simulink model "RWCday13experimentsPWM"  (R2023a)
settings: Solver=ode45  StartTime=0.0  StopTime=100  MaxStep=0.01  RelTol=1e-3
model workspace (MAT data in the model file):
  J = Simulink.Parameter
  J.Value = [0.0067  0  0; 0  0.033  0; 0  0  0.033]
  J.DataType = 'auto'
  J.Complexity = 'real'
  J.Dimensions = [3 3]
  Jscinv = Simulink.Parameter
  Jscinv.DataType = 'auto'
  Jscinv.Complexity = 'real'
  Jscinv.Dimensions = [0 0]
  Td = Simulink.Parameter
  Td.Value = 8.6e-07
  Td.DataType = 'auto'
  Td.Complexity = 'real'
  Td.Dimensions = [1 1]
  Var = 0
  Z = Simulink.Parameter
  Z.DataType = 'auto'
  Z.Complexity = 'real'
  Z.Dimensions = [0 0]
  c = Simulink.Parameter
  c.Value = 20
  c.DataType = 'auto'
  c.Complexity = 'real'
  c.Dimensions = [1 1]
  jw = Simulink.Parameter
  jw.Value = [0.0007  0  0  0; 0  0.0007  0  0; 0  0  0.0007  0; 0  0  0  0.0007]
  jw.DataType = 'auto'
  jw.Complexity = 'real'
  jw.Dimensions = [4 4]
  k = Simulink.Parameter
  k.Value = 0.4
  k.DataType = 'auto'
  k.Complexity = 'real'
  k.Dimensions = [1 1]
  qd = Simulink.Parameter
  qd.Value = [0.752218554293 -0.515629926073 -0.398665163699 -0.0967425096225]
  qd.Description = 'Desired Quaternion'
  qd.DataType = 'auto'
  qd.Complexity = 'real'
  qd.Dimensions = [1 4]
  qd1 = Simulink.Parameter
  qd1.Value = [0; 0; 0; 1]
  qd1.DataType = 'auto'
  qd1.Complexity = 'real'
  qd1.Dimensions = [4 1]
libraries: aerolibutil x3, matrix_library x3, slpidlib x1, dspinverses x1, simulink x1, sharedtransform x1
settings Model: Creator=fatho  LastModifiedBy=fatho
settings SolverCC: ShapePreserveControl=EnableAll

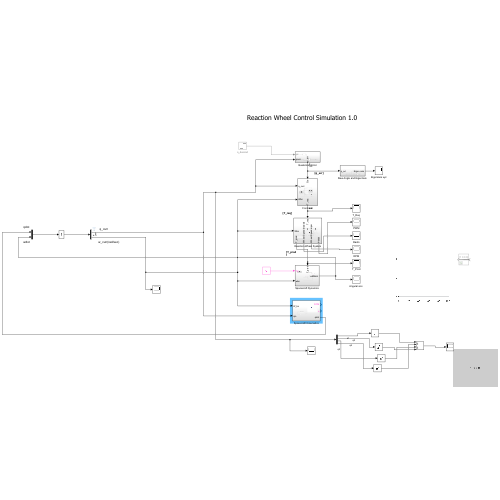
[thumbnail: Simulink's stored preview of the top-level diagram]
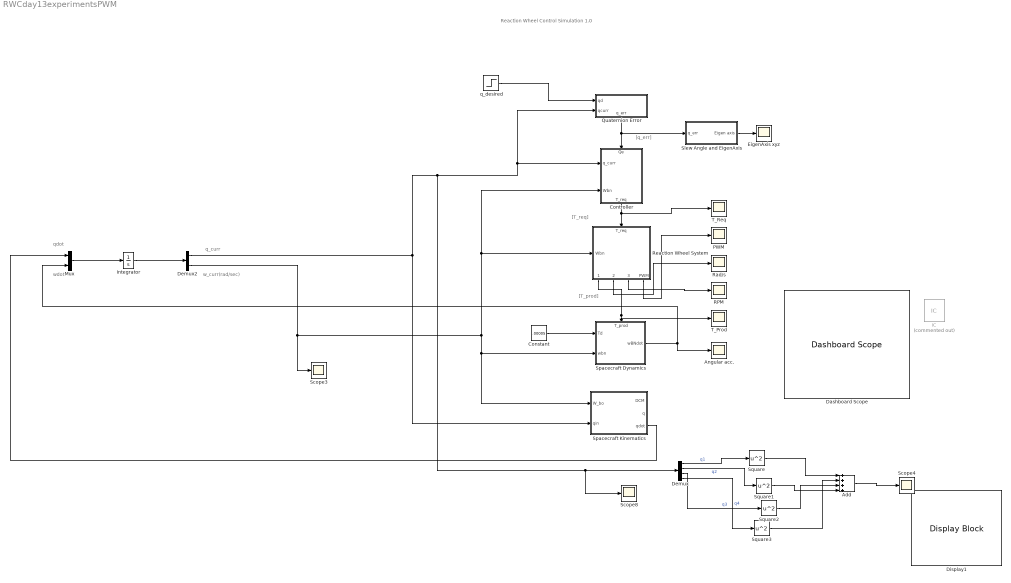
== system RWCday13experimentsPWM ==
  note: wdot
  note: qdot
  note: [T_prod]
  note: [T_req]
  note: Reaction Wheel Control Simulation 1.0
  note: [q_err]
  note: q_curr
  note: w_curr(rad/sec)
  Add : Sum  Inputs=++++
  Angular acc. : Scope
  Constant : Constant  Value=.00005
  Controller : Subsystem
      settings: PortSchema="{\"entries\":[{\"content\":{\"sides\":[{\"content\":{\"connectorIds\":[\"In1\",\"In2\"]},\"type\":\"ConnectorPlacement.EquallySpacedRectSide\",\"uuid\":\"a2df5b41-9ef4-4969-80d2-7b09358407cc\"},{\"content\":{\"side\":\"RIGHT\"},\"type\":\"ConnectorPlacement.EquallySpacedRectSide\",\"uuid\":\"1e6ea160-360b-4529-9fd4-0e8e5500d5a4\"},{\"content\":{\"connectorIds\":[\"In3\"],\"side\":\"TOP\"},\"type\":\"ConnectorPlacement.EquallySpacedRectSide\",\"uuid\":\"8a8b16cc-0742-4909-a1b2-448642d5ccb2\"},{\"content\":{\"connectorIds\":[\"Out1\"],\"side\":\"BOTTOM\"},\"type\":\"ConnectorPlacement.EquallySpacedRectSide\",\"uuid\":\"1d8cf4c9-9e7c-4c9b-9083-d12b460b5772\"}]},\"type\":\"ConnectorPlacement.EquallySpacedConnector\",\"uuid\":\"7465d7f1-526d-43a2-818b-495d95f51981\"}],\"packageUris\":[\"http://schema.mathworks.com/mf0/Connector/R2020b\"],\"version\":\"1.0\"}"
  Dashboard Scope : DashboardScope
  Demux : Demux  Outputs=[1 1 1 1]
  Demux2 : Demux  Outputs=[4 3]
  Display1 : DisplayBlock  LabelPosition=Hide  Transparency=1
  EigenAxis xyz : Scope
  IC : InitialCondition  Commented=on  Value=[1 0 0 0]
  Integrator : Integrator  InitialCondition=[0;0;1;0; 1; 2; 0]  UpperSaturationLimit=1  LowerSaturationLimit=-1  ContinuousStateAttributes='quaterninion'
  Mux : Mux  Inputs=2
  PWM : Scope
  Quaternion Error : Subsystem
      settings: PortSchema="{\"entries\":[{\"content\":{\"sides\":[{\"content\":{\"connectorIds\":[\"In1\",\"In2\"]},\"type\":\"ConnectorPlacement.EquallySpacedRectSide\",\"uuid\":\"2003ebe1-c813-4308-941a-f0b0b97b1ef5\"},{\"content\":{\"side\":\"RIGHT\"},\"type\":\"ConnectorPlacement.EquallySpacedRectSide\",\"uuid\":\"4198199e-7f1d-471e-ae3c-0ca36f291b1d\"},{\"content\":{\"side\":\"TOP\"},\"type\":\"ConnectorPlacement.EquallySpacedRectSide\",\"uuid\":\"ffd6eb4d-f38c-4a17-8c11-c75de219e95d\"},{\"content\":{\"connectorIds\":[\"Out1\"],\"side\":\"BOTTOM\"},\"type\":\"ConnectorPlacement.EquallySpacedRectSide\",\"uuid\":\"7f2c968e-4136-4aca-aa2f-c2c22e58ce6d\"}]},\"type\":\"ConnectorPlacement.EquallySpacedConnector\",\"uuid\":\"d5f6105b-4b4b-42e9-a540-1d01abfad53c\"}],\"packageUris\":[\"http://schema.mathworks.com/mf0/Connector/R2020b\"],\"version\":\"1.0\"}"
  RPM : Scope
  Rad/s : Scope
  Reaction Wheel System : Subsystem
      settings: PortSchema="{\"entries\":[{\"content\":{\"sides\":[{\"content\":{\"connectorIds\":[\"In1\"]},\"type\":\"ConnectorPlacement.EquallySpacedRectSide\",\"uuid\":\"5c21a421-5ce3-4a1e-942c-9be5be815241\"},{\"content\":{\"side\":\"RIGHT\"},\"type\":\"ConnectorPlacement.EquallySpacedRectSide\",\"uuid\":\"ff507b31-edec-4a81-bae3-4543f488c8f2\"},{\"content\":{\"connectorIds\":[\"In2\"],\"side\":\"TOP\"},\"type\":\"ConnectorPlacement.EquallySpacedRectSide\",\"uuid\":\"a44d1fcc-f7cf-4923-a5fc-67e2f5455ac0\"},{\"content\":{\"connectorIds\":[\"Out1\",\"Out2\",\"Out3\",\"Out4\"],\"side\":\"BOTTOM\"},\"type\":\"ConnectorPlacement.EquallySpacedRectSide\",\"uuid\":\"b5c7e00e-dd71-4730-b01d-93b40542af68\"}]},\"type\":\"ConnectorPlacement.EquallySpacedConnector\",\"uuid\":\"3b9b0451-9935-4416-a2af-3f91e1247ebd\"}],\"packageUris\":[\"http://schema.mathworks.com/mf0/Connector/R2020b\"],\"version\":\"1.0\"}"
  Scope3 : Scope
  Scope4 : Scope
  Scope8 : Scope
  "Slew Angle and EigenAxis " : Subsystem
  Spacecraft Dynamics : Subsystem
      settings: PortSchema="{\"entries\":[{\"content\":{\"sides\":[{\"content\":{\"connectorIds\":[\"In1\",\"In2\"]},\"type\":\"ConnectorPlacement.EquallySpacedRectSide\",\"uuid\":\"a2df5b41-9ef4-4969-80d2-7b09358407cc\"},{\"content\":{\"connectorIds\":[\"Out1\"],\"side\":\"RIGHT\"},\"type\":\"ConnectorPlacement.EquallySpacedRectSide\",\"uuid\":\"1e6ea160-360b-4529-9fd4-0e8e5500d5a4\"},{\"content\":{\"connectorIds\":[\"In3\"],\"side\":\"TOP\"},\"type\":\"ConnectorPlacement.EquallySpacedRectSide\",\"uuid\":\"8a8b16cc-0742-4909-a1b2-448642d5ccb2\"}]},\"type\":\"ConnectorPlacement.EquallySpacedConnector\",\"uuid\":\"7465d7f1-526d-43a2-818b-495d95f51981\"}],\"packageUris\":[\"http://schema.mathworks.com/mf0/Connector/R2020b\"],\"version\":\"1.0\"}"
  Spacecraft Kinematics : Subsystem
  Square{,1..3} (4 alike) : Math  Operator=square
  T_Prod : Scope
  T_Req : Scope
  q_desired : Step  Time=0  Before=[0; -1; 0; 0]  After=[0; 0; sqrt(2)/2; sqrt(2)/2]  SampleTime=0
  wires:
  Constant/1 -> Spacecraft Dynamics/1(Td)
  Demux/2 -> Square1/1  "q2"
  Demux/1 -> Square/1  "q1"
  Demux/3 -> Square2/1  "q3"
  Demux/4 -> Square3/1  "q4"
  Demux2/2 -> Spacecraft Kinematics/1(W_bo), Spacecraft Dynamics/2(wbn), Reaction Wheel System/1(Wbn), Controller/2(Wbn), Scope3/1
  Spacecraft Kinematics/3(qdot) -> Mux/1
  Square/1 -> Add/1
  Square1/1 -> Add/4
  Square2/1 -> Add/3
  Square3/1 -> Add/2
  Add/1 -> Scope4/1
  Mux/1 -> Integrator/1
  Integrator/1 -> Demux2/1
  Spacecraft Dynamics/1(wBNdot) -> Mux/2, Angular acc./1
  Demux2/1 -> Spacecraft Kinematics/2(qin), Scope8/1, Demux/1, Quaternion Error/2(qcurr), Controller/1(q_curr)
  Controller/1(T_req) -> Reaction Wheel System/2(T_req), T_Req/1
  Reaction Wheel System/1(T_prod) -> Spacecraft Dynamics/3(T_prod), T_Prod/1
  q_desired/1 -> Quaternion Error/1(qd)
  Quaternion Error/1(q_err) -> Controller/3(Qe), "Slew Angle and EigenAxis "/1(q_err)
  Reaction Wheel System/2(Wheel Speeds rads/s) -> Rad/s/1
  Reaction Wheel System/3(Wheel Speeds rpm) -> RPM/1
  "Slew Angle and EigenAxis "/1(Eigen axis) -> EigenAxis xyz/1
  Reaction Wheel System/4(PWM) -> PWM/1

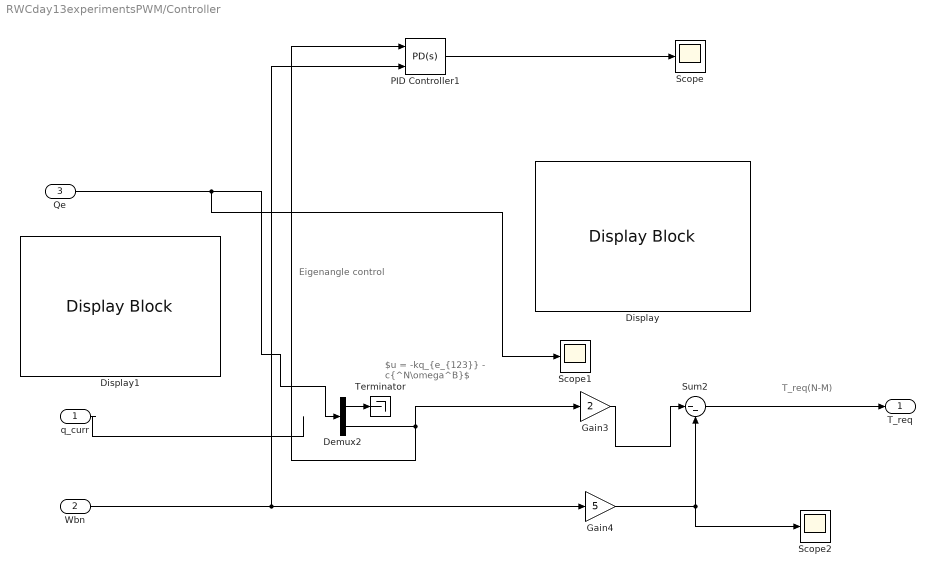
== system RWCday13experimentsPWM/Controller ==
  note: T_req(N-M)
  note: Eigenangle control
  note: $u = -kq_{e_{123}} - c{^N\omega^B}$
  q_curr : Inport
  Wbn : Inport  Port=2
  Qe : Inport  Port=3
  Demux2 : Demux  Outputs=[1 3]
  Display : DisplayBlock  LabelPosition=Hide  Transparency=1
  Display1 : DisplayBlock  LabelPosition=Hide  Transparency=1
  Gain3 : Gain  Gain=2
  Gain4 : Gain  Gain=5
  PID Controller1 : slpidlib/PID Controller  Controller=PD  Form=Parallel  TimeDomain=Continuous-time  UseExternalTs=off  SampleTime=-1  IntegratorMethod=Forward Euler  FilterMethod=Forward Euler  ControllerParametersSource=internal  P=5  I=1  UseKiTs=off  D=55  N=100  UseFilter=on  TunerSelectOption=Transfer Function Based (PID Tuner App)  InitialConditionSource=external  InitialConditionForIntegrator=0  InitialConditionForFilter=0  DifferentiatorICPrevScaledInput=0  ExternalReset=none  TrackingMode=off  Kt=1  LimitOutput=off  SatLimitsSource=internal  UpperSaturationLimit=inf  LowerSaturationLimit=-inf  LinearizeAsGain=on  AntiWindupMode=none  Kb=1  LimitIntegrator=off  UpperIntegratorSaturationLimit=inf  LowerIntegratorSaturationLimit=-inf  POutMin=[]  POutMax=[]  IOutMin=[]  IOutMax=[]  DOutMin=[]  DOutMax=[]  NOutMin=[]  NOutMax=[]  SumOutMin=[]  SumOutMax=[]  SaturationOutMin=[]  SaturationOutMax=[]  PParamMin=[]  PParamMax=[]  IParamMin=[]  IParamMax=[]  DParamMin=[]  DParamMax=[]  NParamMin=[]  NParamMax=[]  KbParamMin=[]  KbParamMax=[]  KtParamMin=[]  KtParamMax=[]  KbOutMin=[]  KbOutMax=[]  KtOutMin=[]  KtOutMax=[]  IntegratorOutMin=[]  IntegratorOutMax=[]  FilterOutMin=[]  FilterOutMax=[]  SumI1OutMin=[]  SumI1OutMax=[]  SumI2OutMin=[]  SumI2OutMax=[]  SumI3OutMin=[]  SumI3OutMax=[]  SumI4OutMin=[]  SumI4OutMax=[]  SumDOutMin=[]  SumDOutMax=[]  DifferentiatorOutMin=[]  DifferentiatorOutMax=[]  FilterDiffOutCoefMin=[]  FilterDiffOutCoefMax=[]  ReciprocalOutMin=[]  ReciprocalOutMax=[]  SumDenOutMin=[]  SumDenOutMax=[]  SumNumOutMin=[]  SumNumOutMax=[]  DivideOutMin=[]  DivideOutMax=[]  UdiffTsProdOutMin=[]  UdiffTsProdOutMax=[]  NTsProdOutMin=[]  NTsProdOutMax=[]  UintegralTsProdOutMin=[]  UintegralTsProdOutMax=[]  UngainTsProdOutMin=[]  UngainTsProdOutMax=[]  ClampingZeroOutDataTypeStr=Inherit: Inherit via back propagation  ClampingZeroOutMin=[]  ClampingZeroOutMax=[]  FilterDenConstantOutDataTypeStr=Inherit: Inherit via back propagation  FilterDenConstantOutMin=[]  FilterDenConstantOutMax=[]  PCopyOutDataTypeStr=Inherit: Inherit via back propagation  PCopyOutMin=[]  PCopyOutMax=[]  NCopyOutDataTypeStr=Inherit: Inherit via back propagation  NCopyOutMin=[]  NCopyOutMax=[]  IntegratorContinuousStateAttributes=''  IntegratorStateMustResolveToSignalObject=off  IntegratorRTWStateStorageClass=Auto  FilterContinuousStateAttributes=''  FilterStateMustResolveToSignalObject=off  FilterRTWStateStorageClass=Auto  ParallelPVariant=InternalParameters  IdealPVariant=Disabled  IVariant=Disabled  DVariant=InternalParameters  IntegratorVariant=Disabled  SatVariant=Disabled  AWVariant=Disabled  PCopyVariant=Disabled  TRVariant=Disabled  FdbkBlocksVariant=Forward  IdealPFdbkVariant=Disabled  SatFdbkVariant=Disabled  DerivativeFilterVariant=ContFilter  NVariant=InternalParameters  NCopyVariant=Disabled  FilterICVariant=ExternalICs  IntegratorICVariant=Disabled  ExternalResetVariant=Disabled  TRSumVariant=Passthrough  SumFdbkVariant=Disabled  SumVariant=Sum_PD  TsampFilterVariant=InternalTs  TsampNgainVariant=Passthrough  TsampIntegralVariant=Disabled_SignalSpec  ExternalSaturationOutDataTypeStr=Inherit: Same as second input
  Scope : Scope
  Scope1 : Scope
  Scope2 : Scope
  Sum2 : Sum  Inputs=|--
  Terminator : Terminator
  T_req : Outport
  wires:
  Gain3/1 -> Sum2/1
  Wbn/1 -> Gain4/1, PID Controller1/2
  Gain4/1 -> Sum2/2, Scope2/1
  Demux2/2 -> PID Controller1/1, Gain3/1
  Sum2/1 -> T_req/1
  Qe/1 -> Scope1/1, Demux2/1
  q_curr/1 -> ?
  Demux2/1 -> Terminator/1
  PID Controller1/1 -> Scope/1

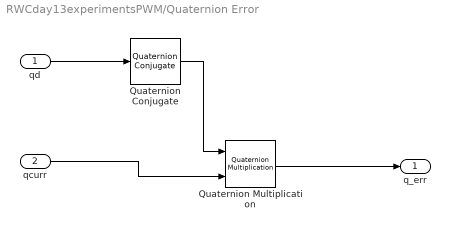
== system RWCday13experimentsPWM/Quaternion Error ==
  qd : Inport
  qcurr : Inport  Port=2
  Quaternion Conjugate : aerolibutil/Quaternion Conjugate
  Quaternion Multiplication : aerolibutil/Quaternion Multiplication
  q_err : Outport
  wires:
  qd/1 -> Quaternion Conjugate/1
  Quaternion Conjugate/1 -> Quaternion Multiplication/1
  qcurr/1 -> Quaternion Multiplication/2
  Quaternion Multiplication/1 -> q_err/1

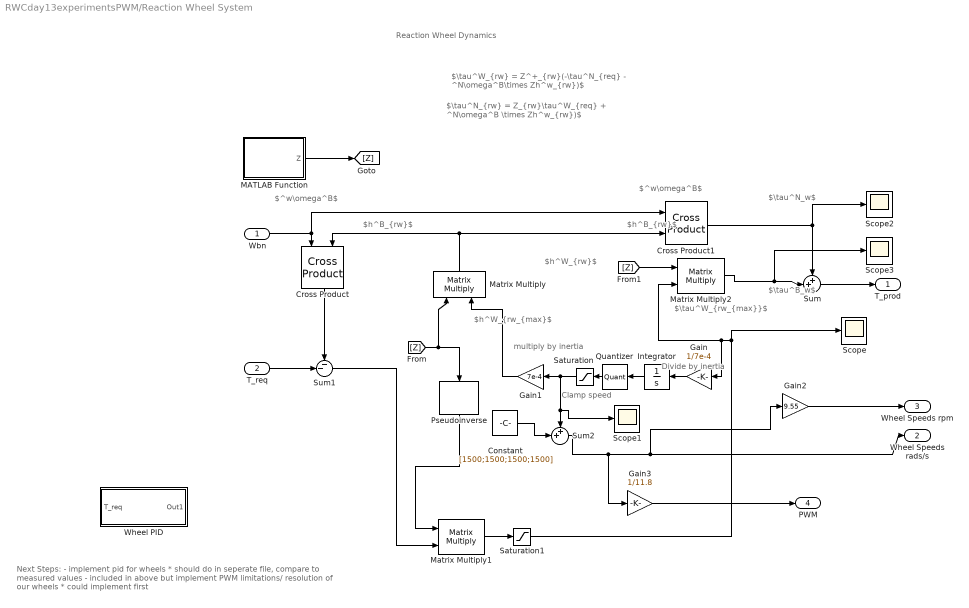
== system RWCday13experimentsPWM/Reaction Wheel System ==
  note: Next Steps:
      | - implement pid for wheels
      | 	* should do in seperate file, compare to measured values
      | - included in above but implement PWM limitations/ resolution of our wheels
      | 	* could implement first
  note: multiply by inertia
  note: Clamp speed
  note: Divide by inertia
  note: $\tau^B_w$
  note: $h^B_{rw}$
  note: $^w\omega^B$
  note: $\tau^W_{rw} = Z^+_{rw}(-\tau^N_{req} - ^N\omega^B\times Zh^w_{rw})$
  note: Reaction Wheel Dynamics
  note: $\tau^N_{rw} = Z_{rw}\tau^W_{req} + ^N\omega^B \times Zh^w_{rw})$
  note: $^w\omega^B$
  note: $h^B_{rw}$
  note: $\tau^N_w$
  note: $\tau^W_{rw_{max}}$
  note: $h^W_{rw}$
  note: $h^W_{rw_{max}$
  Wbn : Inport
  T_req : Inport  Port=2
  Constant : Constant  Value=[1500;1500;1500;1500]
  Cross Product : matrix_library/Cross Product
  Cross Product1 : matrix_library/Cross Product
  Gain : Gain  Gain=1/7e-4
  Gain1 : Gain  Gain=7e-4
  Gain2 : Gain  Gain=9.55
  Gain3 : Gain  Gain=1/11.8
  Integrator : Integrator
  MATLAB Function : MATLAB Function  TreatAsAtomicUnit=on
  Matrix Multiply : Product  Multiplication=Matrix(*)
  Matrix Multiply1 : Product  Multiplication=Matrix(*)
  Matrix Multiply2 : Product  Multiplication=Matrix(*)
  Pseudoinverse : dspinverses/Pseudoinverse  wanterr=off  SimulateUsing=Interpreted execution
  Quantizer : Quantizer  QuantizationInterval=11.8
  Saturation : Saturate  UpperLimit=1500  LowerLimit=-1500
  Saturation1 : Saturate  UpperLimit=.003  LowerLimit=-.003
  Scope{,1..3} (4 alike) : Scope
  Sum : Sum  Inputs=++|
  Sum1 : Sum  Inputs=--|
  Sum2 : Sum  Inputs=++|
  Wheel PID : Subsystem
  T_prod : Outport
  Wheel Speeds rads/s : Outport  Port=2
  Wheel Speeds rpm : Outport  Port=3
  PWM : Outport  Port=4
  wires:
  Pseudoinverse/1 -> Matrix Multiply1/1
  MATLAB Function/1(Z) -> [Z]
  [Z] -> Matrix Multiply/1, Pseudoinverse/1
  Wbn/1 -> Cross Product1/1, Cross Product/1
  [Z] -> Matrix Multiply2/1
  Matrix Multiply1/1 -> Saturation1/1
  Matrix Multiply/1 -> Cross Product1/2, Cross Product/2
  Cross Product1/1 -> Sum/1, Scope2/1
  Sum/1 -> T_prod/1
  T_req/1 -> Sum1/2
  Cross Product/1 -> Sum1/1
  Sum1/1 -> Matrix Multiply1/2
  Saturation/1 -> Gain1/1, Scope1/1, Sum2/1
  Gain1/1 -> Matrix Multiply/2
  Gain2/1 -> Wheel Speeds rpm/1
  Saturation1/1 -> Scope/1, Matrix Multiply2/2, Gain/1
  Integrator/1 -> Quantizer/1
  Gain/1 -> Integrator/1
  Constant/1 -> Sum2/2
  Sum2/1 -> Gain3/1, Gain2/1, Wheel Speeds rads/s/1
  Matrix Multiply2/1 -> Scope3/1, Sum/2
  Quantizer/1 -> Saturation/1
  Gain3/1 -> PWM/1

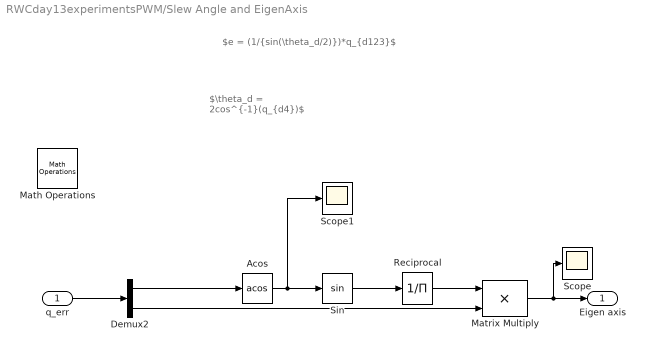
== system RWCday13experimentsPWM/Slew Angle and EigenAxis  ==
  note: $\theta_d = 2cos^{-1}(q_{d4})$
  note: $e = (1/{sin(\theta_d/2)})*q_{d123}$
  q_err : Inport
  Acos : Trigonometry  Operator=acos
  Demux2 : Demux  Outputs=[1 3]
  Math Operations : simulink/Quick Insert/Math Operations  SystemSampleTime=-1  VariantActivationTime=update diagram  Latency=0  AutoFrameSizeCalculation=off
  Matrix Multiply : Product
  Reciprocal : Product  Inputs=/
  Scope : Scope
  Scope1 : Scope
  Sin : Trigonometry
  Eigen axis : Outport
  wires:
  q_err/1 -> Demux2/1
  Demux2/1 -> Acos/1
  Acos/1 -> Scope1/1, Sin/1
  Sin/1 -> Reciprocal/1
  Reciprocal/1 -> Matrix Multiply/1
  Demux2/2 -> Matrix Multiply/2
  Matrix Multiply/1 -> Scope/1, Eigen axis/1

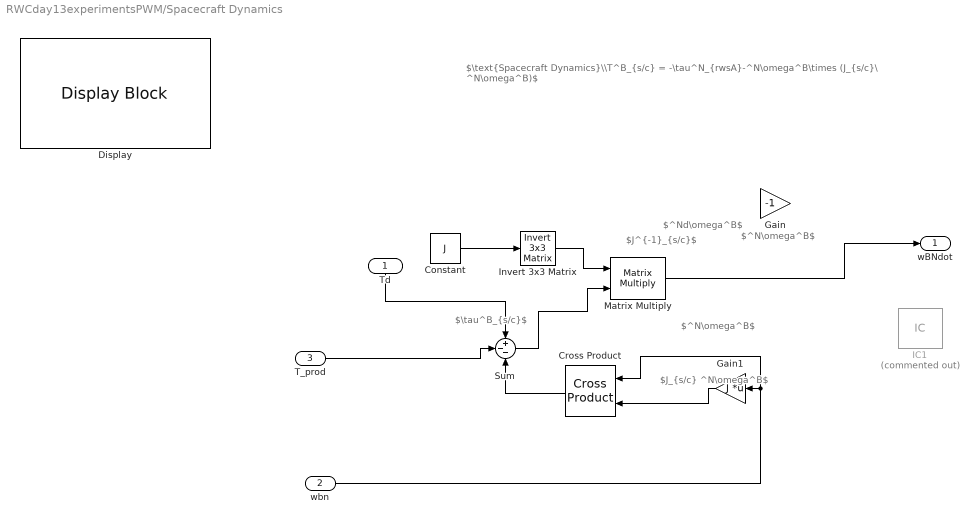
== system RWCday13experimentsPWM/Spacecraft Dynamics ==
  note: $^Nd\omega^B$
  note: $J^{-1}_{s/c}$
  note: $\tau^B_{s/c}$
  note: $\text{Spacecraft Dynamics}\\T^B_{s/c} = -\tau^N_{rwsA}-^N\omega^B\times (J_{s/c}\ ^N\omega^B)$
  note: $^N\omega^B$
  note: $^N\omega^B$
  note: $J_{s/c} ^N\omega^B$
  Td : Inport
  wbn : Inport  Port=2
  T_prod : Inport  Port=3
  Constant : Constant  Value=J
  Cross Product : matrix_library/Cross Product
  Display : DisplayBlock  LabelPosition=Hide  Transparency=1
  Gain : Gain  Gain=-1
  Gain1 : Gain  Gain=J  Multiplication=Matrix(K*u)
  IC1 : InitialCondition  Commented=on  Value=[0; 2; 0]
  Invert 3x3 Matrix : aerolibutil/Invert  3x3 Matrix
  Matrix Multiply : Product  Multiplication=Matrix(*)
  Sum : Sum  Inputs=+--
  wBNdot : Outport
  wires:
  Td/1 -> Sum/1
  T_prod/1 -> Sum/2
  Cross Product/1 -> Sum/3
  Gain1/1 -> Cross Product/2
  Sum/1 -> Matrix Multiply/2
  Constant/1 -> Invert 3x3 Matrix/1
  Invert 3x3 Matrix/1 -> Matrix Multiply/1
  Matrix Multiply/1 -> wBNdot/1
  wbn/1 -> Cross Product/1, Gain1/1

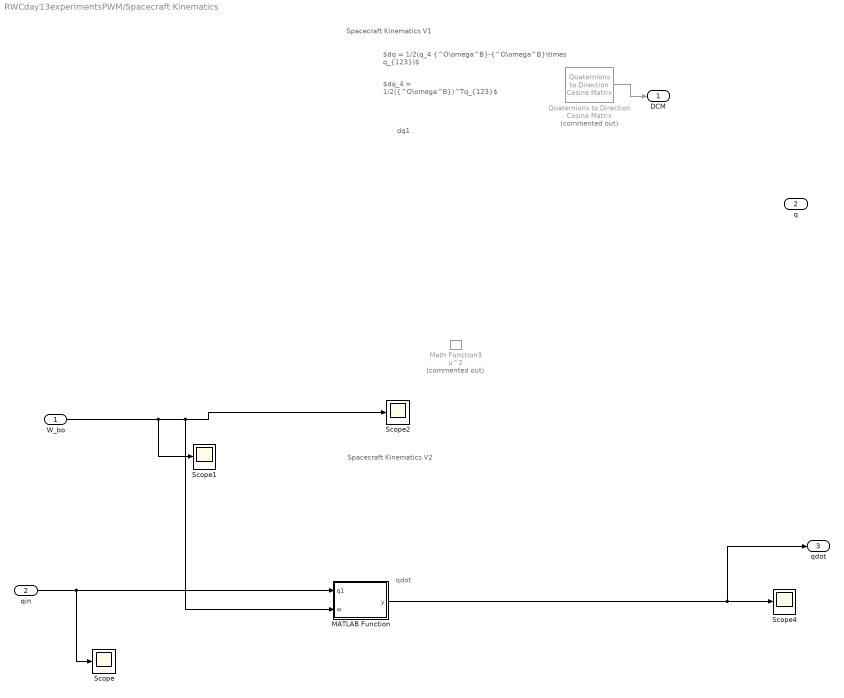
== system RWCday13experimentsPWM/Spacecraft Kinematics ==
  note: qdot
  note: Spacecraft Kinematics V2
  note: dq1
  note: Spacecraft Kinematics V1
  note: $dq_4 = 1/2({^O\omega^B})^Tq_{123}$
  note: $dq = 1/2(q_4 {^O\omega^B}-{^O\omega^B}\times q_{123})$
  W_bo : Inport
  qin : Inport  Port=2
  MATLAB Function : MATLAB Function  TreatAsAtomicUnit=on
  Math Function3 : Math  Commented=on  Operator=square
  Quaternions to Direction Cosine Matrix : sharedtransform/Quaternions to  Direction Cosine Matrix  Commented=on  aMode=aMode
      settings: LibrarySourceBlock=|
      | aerolibtransform2/Quaternions to
      | Direction Cosine Matrix
  Scope{,1..2,4} (4 alike) : Scope
  DCM : Outport
  q : Outport  Port=2  PortDimensions=[1 4]
  qdot : Outport  Port=3  PortDimensions=[4 1]
  wires:
  Quaternions to Direction Cosine Matrix/1 -> DCM/1
  W_bo/1 -> Scope1/1, MATLAB Function/2(w), Scope2/1
  MATLAB Function/1(y) -> qdot/1, Scope4/1
  qin/1 -> Scope/1, MATLAB Function/1(q1)

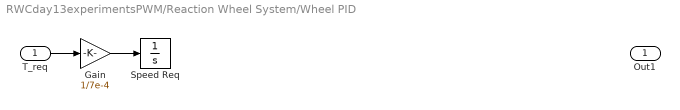
== system RWCday13experimentsPWM/Reaction Wheel System/Wheel PID ==
  T_req : Inport
  Gain : Gain  Gain=1/7e-4
  Speed Req : Integrator
  Out1 : Outport
  wires:
  Gain/1 -> Speed Req/1
  T_req/1 -> Gain/1

== matlab function RWCday13experimentsPWM/Spacecraft Kinematics/MATLAB Function ==
  data: q1 input; w input; y output
function y = fcn(q1, w)
w1 = w(1);
w2 = w(2);
w3 = w(3);

W = [0 -w1 -w2 -w3; w1 0 w3 -w2; w2 -w3 0 w1; w3 w2 -w1 0];

q11 = q1(1)*0 -w1*q1(2) -w2*q1(3) -w3*q1(4);
q12 = q1(1)*w1 + 0*q1(2) - w3*q1(3) +w2*q1(4);
q13 = q1(1)*w2 +w3*q1(2) + 0*q1(3) - w1*q1(4);
q14 = q1(1)*w3 - w2*q1(2) +w1*q1(3) + 0*q1(4);

u1 = .5 * [q11; q12; q13; q14];
u2 = .5 * W * q1;
y = u2;

== matlab function RWCday13experimentsPWM/Reaction Wheel System/MATLAB Function ==
  data: Z output
function Z = fcn

Z = 1/sqrt(3)*[sqrt(2) 0 -sqrt(2) 0; 0 sqrt(2) 0 -sqrt(2); 1 1 1 1];
